simulink model "ES101A_DiagcMgr"  (R2013b)
settings: Solver=ode45  StartTime=0.0  StopTime=0.44  RelTol=1e-3
values from neighbouring files (symbols this model uses):
  BrdgVltg = DataDict.IpSignal    [ES101A_DiagcMgr_DataDict.m]
  DEM_CLEAR_PENDING = DataDict.Constant    [ES101A_DiagcMgr_DataDict.m]
  DEM_DTC_GROUP_ALL_DTCS = DataDict.Constant    [ES101A_DiagcMgr_DataDict.m]
  DFTAGICNTR_CNT_U08 = DataDict.Constant    [ES101A_DiagcMgr_DataDict.m]
  DIAGCMGR_NTCINFOSTSTESTFAILD_CNT_U08 = DataDict.Constant    [ES101A_DiagcMgr_DataDict.m]
  DIAGCMGR_NTCINFOSTSTESTFAILDTHISIGNCYC_CNT_U08 = DataDict.Constant    [ES101A_DiagcMgr_DataDict.m]
  DIAGCMGR_NTCINFOSTSTESTNOTCMPLTHISIGNCYC_CNT_U08 = DataDict.Constant    [ES101A_DiagcMgr_DataDict.m]
  DiagcMgrFltResp = DataDict.Calibration    [ES101A_DiagcMgr_DataDict.m]
  DiagcMgrNtcFltAry = DataDict.NVM    [ES101A_DiagcMgr_DataDict.m]
  DIAGCSTSCTRLDSHTDWNFLTPRSNT_CNT_U16 = DataDict.Constant    [ES101A_DiagcMgr_DataDict.m]
  DIAGCSTSDFTHWAG_CNT_U16 = DataDict.Constant    [ES101A_DiagcMgr_DataDict.m]
  DIAGCSTSDFTHWAGSERLCOMEXPRTVAL_CNT_U16 = DataDict.Constant    [ES101A_DiagcMgr_DataDict.m]
  DIAGCSTSDFTVEHSPD_CNT_U16 = DataDict.Constant    [ES101A_DiagcMgr_DataDict.m]
  DIAGCSTSININVAL_CNT_U16 = DataDict.Constant    [ES101A_DiagcMgr_DataDict.m]
  DIAGCSTSIVTR1INACTV_CNT_U16 = DataDict.Constant    [ES101A_DiagcMgr_DataDict.m]
  DIAGCSTSIVTR2INACTV_CNT_U16 = DataDict.Constant    [ES101A_DiagcMgr_DataDict.m]
  DIAGCSTSLIMDTPRFMNC_CNT_U16 = DataDict.Constant    [ES101A_DiagcMgr_DataDict.m]
  DIAGCSTSRAMPTOZEROFLTPRSNT_CNT_U16 = DataDict.Constant    [ES101A_DiagcMgr_DataDict.m]
  DIAGCSTSWHLIMBREJCTNDI_CNT_U16 = DataDict.Constant    [ES101A_DiagcMgr_DataDict.m]
  DTCIDXSTSFAIL_CNT_U08 = DataDict.Constant    [ES101A_DiagcMgr_DataDict.m]
  DTCIDXSTSNONTC_CNT_U08 = DataDict.Constant    [ES101A_DiagcMgr_DataDict.m]
  DTCIDXSTSNORES_CNT_U08 = DataDict.Constant    [ES101A_DiagcMgr_DataDict.m]
  DTCIDXSTSPASS_CNT_U08 = DataDict.Constant    [ES101A_DiagcMgr_DataDict.m]
  DTCIDXSTSUPDCFMD_CNT_U08 = DataDict.Constant    [ES101A_DiagcMgr_DataDict.m]
  ELECGLBPRM_IVTRCNT_CNT_U08 = DataDict.ConfigParam    [ES101A_DiagcMgr_DataDict.m]
  FLTINJ_DIAGCMGR_DIAGCSTSIVTR1INACTV = DataDict.Constant    [ES101A_DiagcMgr_DataDict.m]
  FLTINJ_DIAGCMGR_DIAGCSTSIVTR2INACTV = DataDict.Constant    [ES101A_DiagcMgr_DataDict.m]
  HwTq = DataDict.IpSignal    [ES101A_DiagcMgr_DataDict.m]
  IgnCntr = DataDict.IpSignal    [ES101A_DiagcMgr_DataDict.m]
  MAXDEBCNTRVAL_CNT_S16 = DataDict.Constant    [ES101A_DiagcMgr_DataDict.m]
  MAXRAMPRATE_ULSPERSEC_F32 = DataDict.Constant    [ES101A_DiagcMgr_DataDict.m]
  MINDEBCNTRVAL_CNT_S16 = DataDict.Constant    [ES101A_DiagcMgr_DataDict.m]
  MINRAMPRATE_ULSPERSEC_F32 = DataDict.Constant    [ES101A_DiagcMgr_DataDict.m]
  SCAMOTTQCMDTOONE_ULS_F32 = DataDict.Constant    [ES101A_DiagcMgr_DataDict.m]
  SCAMOTTQCMDTOZERO_ULS_F32 = DataDict.Constant    [ES101A_DiagcMgr_DataDict.m]
  SysSt = DataDict.IpSignal    [ES101A_DiagcMgr_DataDict.m]
  VehSpd = DataDict.IpSignal    [ES101A_DiagcMgr_DataDict.m]
undefined symbols (not defined in the file or in its folder): ActvMotTqCmdSca, ActvRampRate, AgiCntr, Dem_DTCFormatType, Dem_DTCOriginType, Dem_EventStatusType, DiagcData, DiagcMgrNtcMap, DiagcSts, DtcEnaMask, EcuT, HistNtcFltAry, MicroDiagcData, MotTq, NtcNr, NtcNrWithResd1, NtcStInfo, ProxySetNtcData, Sts, SysSt1, TOTNROFDTC_CNT_U08
libraries: simulink x151, FloatToFixd x5, NxtrNvM x4
(part 1 of 13)
settings Model: Creator=NZG49T  LastModifiedBy=nzg49t
settings DataIOCC: SaveFormat=Structure

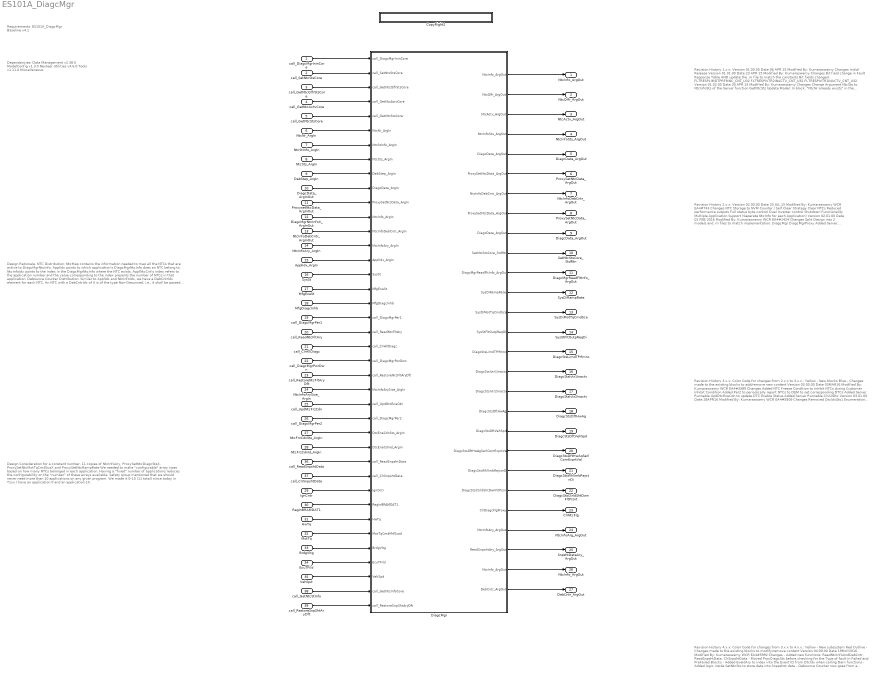
== system ES101A_DiagcMgr ==
  note: Revision History 1.x.x:
      |
      | Version		01.00.00
      | Date 		06 APR 15
      | Modified By: 	Kumaraswamy
      | Changes		Initial Release
      |
      | Version		01.01.00
      | Date 		23 APR 15
      | Modified By: 	Kumaraswamy
      | Changes		Bit field change in Fault Response Table AND update the .m file to match the constants
      | 			Bit fields changed: 	FLTRESPLIMDTPRFMNC_CNT_U32
      | 								FLTRESPIVTR2INACTV_CNT_U32
      | 								FLTRESPIVTR1INACTV_CNT_U32
      |
      | Version		01.02.00
      | Date 		30 APR 15
      | Modified By: 	Kumaraswamy
      | Changes		Change Argument NtcSts to NtcInfoSts of the Server function GetNtcSts
      | 			Update Model: In block, "NtcNr already exists" in the NtcFltAry when NTC fails, update the status byte
      | 			to show test failed bit as SET.
  note: Dependancies:
      |
      |    Data Management v2.38.0
      |    ModelConfig v1.3.0
      |    Nexteer Utilities v4.6.0
      |    Tools v1.11.0
      |    Miscellaneous
  note: Design Rationale:
      |
      | 	NTC Distribution:
      | 		NtcMap contains the information needed to map all the NTCs that are active to DiagcMgrNtcInfo.
      | 		ApplIdx points to which application's DiagcMgrNtcInfo does an NTC belong to.
      | 		NtcInfoIdx points to the index in the DiagcMgrNtcInfo where the NTC exists.
      | 		ApplNtcCnt's index refers to the application number and the value corresponding
      | 			to the index presents the number of NTCs in that application.
      |
      | 	Debounce Counter Distribution:
      | 		Similar to ApplIdx and NtcInfoIdx, we have a DebCntrIdx element for each NTC. An NTC with a DebCntrIdx of 0 is of the type Non-Deounced,
      | 		i.e., it shall be passed with SetNtcSts with NtcSts of either Passd or Faild only.
      | 		An NTC with a DebCntrIdx of Non-Zero is of the type Deounced, i.e., it shall be passed with SetNtcSts with NtcSts of either PrePassd or
      | 		PreFaild only.
      | 		Index 0 is used as a scratch pad for all the NTCs that are of the type Non-Debounced.
      |
      | 	NtcInfo for each application:
      | 		There will be a total of 11 DiagcMgrNtcInfo, one for each application.
      | 		If, for a specific program, we have 4 applications(say 0,3,4,10), each of these 4 applications with have certain number of NTCs in its respective
      | 		DiagcMgrNtcInfo(0,3,4,10). The rest of the DiagcMgrNtcInfo(1,2,5,6,7,8,9) will have just one element with the following default values:
      | 			AgiCntr:		255
      | 			Sts:			0
      | 			NtcStInfo:	0
      | 		Each application has its own array of structures that contains NTCs specific to its application.
      | 		The NTCs in any application will not be modified by any other application.
      |
      | 	DiagcSts, RampRate and Scale:
      | 		Each application will have a DiagcStsX, ProxyPerDiagcStsX and ProxySetNtcDiagcStsX (X is the application number):
      | 			DiagcStsX and ProxySetNtcDiagcStsX will be updated everytime the SetNtcSts function is called from the application.
      |
      | 			Each application makes a call to the DiagcMgrPer2 and clears the ProxyPerDiagcStsX and ProxySetNtcDiagcStsX.
      | 			DiagcMgrPer2 runs through all the NTCs in the application and updates the ProxyPerDiagcStsX with the most recent info
      | 			of all the NTCs that have failed this in this ignition cycle while ProxySetNtcDiagcStsX gets updated along with DiagcStsX
      | 			in the SetNtcSts function if any faults are set during the execution of DiagcMgrPer2.
      |
      | 			At the end of DiagcMgrPer2, DiagcStsX is  set equal to the ORed values of ProxyPerDiagcStsX and ProxySetNtcDiagcStsX
      |
      | 			DiagcMgrDiagcSts is the Word which stores the values that output the reduced performanc flags.
      | 			This value ORs all the DiagcStsX values and outputs the reduced performance flags in the DiagcMgrPer1.
      |
      | 			The same design rationale applies to RampRate  and Motor Torque Command Scale.
      | 			At the end of DiagcMgrPer2, RampRateX is  set to the MAX values of ProxyPerRampRateX and ProxySetNtcRampRateX.
      | 			At the end of DiagcMgrPer2, MotTqCmdScaX is  set to the MIN values of ProxyPerMotTqCmdScaX and ProxySetNtcMotTqCmdScaX.
      |
      | 	DiagcMgrInin:
      | 		DiagcMgrInin function shall be treated like server runnables by each application. An applicaiton shall call
      | 		DiagcMgrInin at initialization once passing the address of DiagcMgrNtcInfo to the DiagcMgr.
      |
      | 	DiagcMgrProxyPer1:
      | 		Each application will call DiagcMgrProxyPer1 at every 10ms interval passing the address of ProxySetNtcDiagcStsX. (X is the application number)
      | 		This is shown in DiagcMgrProxyX model.
      |
      | 	Model to SW Implementation:
      | 		Each NTC is mapped to only one of the DiagcMgrNtcInfo0 through 1DiagcMgrNtcInfo10 which will
      | 		be accessed by a pointer to the array of structure.
      | 		Model uses IF condition to look up the DiagcMgrNtcInfo (0 through 10) and uses the NtcInfoIdx to Index
      | 		into the NtcNr in the DiagcMgrNtcInfo.
      | 		SW implemention could involve using pointers to access the DiagcMgrNtcInfo (0 through 10) and use the
      | 		NtcInfoIdx to Index into the NtcNr in the DiagcMgrNtcInfo.
      |
      | 	Proxy Diagnostic Manager:
      | 		Each application will house a ProxyDiagnosticManager. Whenever a component inside an application calls
      | 		one of the server runnables, the ProxyDiagnosticManager makes a function call to the DiagcMgr and passes
      | 		some additional information of ApplIdx along with NtcNr, NtcSts, DebStep and NtcStInfo.
      |
      | 		The server runnables include DiagcMgrInit, SetNtcSts, GetNtcQlftSts, GetNtcActv and GetNtcSts.
      |
      | 	Handling Motor Control Interrrupts:
      | 		ES101A_v2_x_0 and above assumes that the Motor Control loop cannot set faults (call server runnables of DiagcMgr).
      |
      | 	Setting an NTC:
      | 		ES101A_v2_x_0 and above assumes that the same NTC Number cannot be set in mutilple loops
  note: Design Consideration for a constant number, 11 copies of NtcInfoAry, ProxySetNtcDiagcStsX, ProxySetNtcMotTqCmdScaX and ProxySetNtcRampRate
      |
      | We needed to make "configurable" array sizes based on how many NTCs belonged in each application.
      | Having a "fixed" number of applications reduces the configurability on the "number" of these arrays  available.
      | Safety group mentioned that we should never need more than 10 applications on any given program.
      | We made it 0-10 (11 total) since today in T1xx I have an application 0 and an application 10.
  note: Requirements:
      | ES101A_DiagcMgr Baseline v4.1
  note: Revision History 2.x.x:
      |
      | Version		02.00.00
      | Date 		20 JUL 15
      | Modified By: 	Kumaraswamy
      | WCR		EA4#743
      | Changes		NTC Storage to NVM
      | 			Counter / Self Clear Strategy
      | 			Clear NTCs
      | 			Reduced performance outputs
      | 			Full status byte control
      | 			Dual Inverter control
      | 			Shutdown Functionality
      | 			Multiple Application Support (Seperate NtcInfo for each Application)
      |
      | Version		02.01.00
      | Date 		02 FEB 2016
      | Modified By: 	Kumaraswamy
      | WCR		EA4#1424
      | Changes		Split Design into 2 models and .m files to match implementation:
      | 				DiagcMgr
      | 				DiagcMgrProxy
      | 			Added Server Runnables in DiagcMgr:
      | 				DiagcMgrIninCore
      | 				ClrAllNtc
      | 				RestoreNtcFltAryDft
      | 			Added Server Runnables in DiagcMgrProxy:
      | 				GetDiagcDataApplX
      | 				GetNtcInfoApplX
      | 			DiagcMgrActv Output is removed.
  note: Revision History 4.x.x:
      |
      | Color Code for changes from 3.x.x to 4.x.x.:
      | 	Yellow -  New subsystem
      | 	Red Outline -  Changes made to the existing blocks to modify/remove content
      |
      | Version		04.00.00
      | Date 		19MAY2016
      | Modified By: 	Kumaraswamy
      | WCR		EA4#5992
      | Changes		- Added new functions: ReadNtcInfoAndDebCntr, ReadSnpshtData, ClrSnpshtData
      | 			- Moved ProcDiagcSts before checking for the Type of fault in Failed and PreFailed Blocks
      | 			- Added EveIdAry to index into the Event ID from DtcIdx when calling Dem functions
      | 			- Added logic inside SetNtcSts to store data into Snapshot data
      | 			- Debounce Counter now goes from a negative value to DebStep if a Fail call is made to an NTC
      |
      | Version		04.01.00
      | Date 		16JUN2016
      | Modified By: 	Mohan
      | WCR		EA4#6355
      | Changes		- Added fault injection blocks in DiagcMgrPer1
      |
      | Version		04.02.00
      | Date 		21JUN2016
      | Modified By: 	Kumaraswamy
      | WCR		EA4#6360
      | Changes		- Changed call to the DEM: Clear all DTCs in DiagcMgrPer2
      | 			- Loop counter datatype changed from int32 to int16 in RestoreSnpshtAryDft
      | 			- RestoreSnpshtAryDft and RestoreNtcFltAryDft
      | 			- Changed argument SnpshtDataAry_ArgOut to ReadSnpshtAry_ArgOut of ReadSnpshtData Server Runnable
      | 			- Updated the GetNtcQlfrStsCore, GetNtcStsCore and GetNtcActvCore's default case
      | 			- Added client call GetNtcDebCntrAppIX to read the Debounce Counter of any NTC in any application
      | 			- Created a subgroup to create the snapshot bus to link to requirements
      |
      | Version		04.02.01
      | Date 		29JUN2016
      | Modified By: 	Kumaraswamy
      | WCR		EA4#6458
      | Changes		- Removed Data Type Convert blocks when loading 0s to NvM Block of SnpshtAry in RestoreSnpshtAryDft
      | 			- Added output out of the Default Case Switch Statement in Per2 for all NTCs
      | 			- Added a condition in If to check if DTC Idx is less than or equal to TOTNROFDTC_CNT_U08 in Per2
      | 			- ClrSnpshtData loaded with correct default values
      |
      | Version		04.03.00
      | Date 		15AUG2016
      | Modified By: 	Kumaraswamy
      | WCR		EA4#6904
      | Changes		- PIL Optimizations
      |
      | Version		04.04.00
      | Date 		14SEP2016
      | Modified By: 	Kumaraswamy
      | WCR		EA4#7573
      | Changes		- Overflow condition averted by adding logic in "if condition" inside PreFaild
      | 			- Added logic to return a 0 value of DebCntr for Non Debounced NTCs in the ReadNtcInfoAndDebCntr server runnable
      | 			since all Non Debounced NTCs use the DebCntrIdx of 0 as a scratchpad
      |
      | Version		04.05.00
      | Date 		15NOV2016
      | Modified By: 	Kumaraswamy
      | WCR		EA4#8249
      | Changes		- UpdSnpshtData  logic updated to prevent multiple entries of same NTC being set
      | 			- Added logic to call UpdSnpshtData only once if the NTC transitions from Pass to Fail
      |
      | Version		04.06.00
      | Date 		01DEC2016
      | Modified By: 	Kumaraswamy
      | WCR		EA4#8667
      | Changes		- Added write to Set Ram Block Status in ClrSnpshtData  function after the for loop
  note: Revision History 3.x.x:
      |
      | Color Code for changes from 2.x.x to 3.x.x.:
      | 	Yellow -  New blocks
      | 	Blue -  Changes made to the existing blocks to add/remove new content
      |
      | Version		03.00.00
      | Date 		03MAR16
      | Modified By: 	Kumaraswamy
      | WCR		EA4#3389
      | Changes
      | 			Added NTC Freeze Condition to Inhibit NTCs during Customer Inhibit Condition
      | 			Added Per2 to periodically report NTCs to DEM to set corresponding DTCs
      | 			Added Server Runnable UpdDtcEnaCdn to update DTC Enable Status
      | 			Added Server Runnable ClrAllDtc
      |
      | Version		03.01.00
      | Date 		28APR16
      | Modified By: 	Kumaraswamy
      | WCR		EA4#5509
      | Changes		Removed DtcIdxSts1 Enumeration and replaced it's members with constants since it is used
      | 			only by temp variables
      | 			ReadNtcFltAry's output argument renamed correctly as per .m file
      | 			Comments updated
      | 			Added PIM PrevClrDiagcFlag in the .m file
      |
      | Version		03.02.00
      | Date 		29APR16
      | Modified By: 	Kumaraswamy
      | WCR		EA4#5509
      | Changes		Initialized DtcIdxCurrSts 0th element in the Initialization of Per2
      | 			Matched the PrevClrDtcFlg, ClrDtcFlg, ClrDiagcFlgProxy, PrevClrNtcFlgX to have a DataType of Boolean in .m file
      | 			UpdDtcEnaCdn changed from Rte to NonRte
      |
      | Version		03.03.00
      | Date 		26MAY16
      | Modified By: 	Kumaraswamy
      | WCR		EA4#5907
      | Changes		Updated the description of DtcEnaMask to show the length of the array.
  call_DiagcMgrIninCore : Inport
  call_SetNtcStsCore : Inport  Port=2
  call_GetNtcQlfrStsCore : Inport  RequirementInfo={} %GIDa_139edafb_ed2e_4817_b523_bf8478521829  Port=3
  call_GetNtcActvCore : Inport  Port=4
  call_GetNtcStsCore : Inport  Port=5
  NtcNr_ArgIn : Inport  Port=6
  NtcStInfo_ArgIn : Inport  Port=7
  NtcSts_ArgIn : Inport  Port=8
  DebStep_ArgIn : Inport  Port=9
  DiagcData_ArgInOut : Inport  Port=10
  ProxysetNtcData_ArgInOut : Inport  RequirementInfo={} %GIDa_51b0a352_6025_4132_85e8_dce6b37dec3f  Port=11
  DiagcMgrNtcInfoX_ArgInOut : Inport  Port=12
  NtcInfoDebCntr_ArgInOut : Inport  Port=13
  NtcInfoAry_ArgIn : Inport  Port=14
  ApplIdx_ArgIn : Inport  Port=15
  SysSt : Inport  Port=16
  MfgEnaSt : Inport  Port=17
  MfgDiagcInhb : Inport  RequirementInfo="{'linktype_rmi_doors' '0000c474 (/ESG Group/FDD Module Requirements/EA4 Specific/ES101A_DiagcMgr)' '#ES101A_301' 'true' 'REQ:  ES101A_301' '' } %GIDa_f9f3ee9e_ad90_4a3f_b3fd_4c7a6708a1f3"  Port=18
  call_DiagcMgrPer1 : Inport  Port=19
  call_ReadNtcFltAry : Inport  Port=20
  call_ClrAllDiagc : Inport  Port=21
  call_DiagcMgrPwrDwn : Inport  Port=22
  call_RestoreNtcFltAryDft : Inport  Port=23
  NtcInfoArySize_ArgIn : Inport  Port=24
  call_UpdNtcFrzCdn : Inport  Port=25
  call_DiagcMgrPer2 : Inport  Port=26
  NtcFrzCdnSts_ArgIn : Inport  Port=27
  NtcFrzCdnId_ArgIn : Inport  Port=28
  IgnCntr : Inport  Port=29
  RegInBRAMDAT1 : Inport  Port=30
  HwTq : Inport  Port=31
  MotTq : Inport  Port=32
  BrdgVltg : Inport  Port=33
  EcuTFild : Inport  Port=34
  VehSpd : Inport  Port=35
  call_ReadSnpshtData : Inport  Port=36
  call_ClrSnpshtData : Inport  Port=37
  call_GetNtcStInfo : Inport  Port=38
  call_RestoreSnpShtAryDft : Inport  Port=39
  CopyRight2 : Subsystem  Description=|  mask(Copyright Information){none=on}
      | Copyright info block.                                               
      |                                                                     
      | Place copyright information at the top of every subsystem in design.
      mask prompts: none "No parameters"
      mask help: Place copyright information at the top of every subsystem in design.
      mask Display:
      | NxtrConf = 'Nexteer Confidential';
      | 
      | sys = bdroot; %handle for the current model ("system")
      | first = get_param(sys,'Created');
      | first = first(end-3:end);  %year is last four digits
      | 
      | last = get_param(sys,'LastModifiedDate');
      | if isempty(last)
      |     last = datestr(now,'yyyy');
      | else
      |     last = last(end-3:end);
      | end
      | 
      | if strcmp(first,last)
      |     fprintf('%s -- Copyright %s Nexteer',NxtrConf,first)
      | else
      |     fprintf('%s -- %s%s- %s Nexteer',NxtrConf,char(169),first,last)
      | end
  DiagcMgr : Subsystem
  "NtcInfo_ArgOut " : Outport
  NtcQlfr_ArgOut : Outport  Port=2
  NtcActv_ArgOut : Outport  Port=3
  NtcInfoSts_ArgOut : Outport  Port=4
  "DiagcData_ArgOut " : Outport  Port=5
  "ProxySetNtcData_ArgOut " : Outport  Port=6
  "NtcInfoDebCntr_ArgOut " : Outport  Port=7
  ProxySetNtcData_ArgOut : Outport  Port=8
  DiagcData_ArgOut : Outport  Port=9
  SetNtcStsCore_StdRtn : Outport  Port=10
  DiagcMgrReadFltInfo_ArgOut : Outport  Port=11
  SysDiRampRate : Outport  Port=12
  SysDiMotTqCmdSca : Outport  Port=13
  SysStFltOutpReqDi : Outport  Port=14
  DiagcStsLimdTPrfmnc : Outport  Port=15
  DiagcStsIvtr1Inactv : Outport  Port=16
  DiagcStsIvtr2Inactv : Outport  Port=17
  DiagcStsDftHwAg : Outport  Port=18
  DiagcStsDftVehSpd : Outport  Port=19
  DiagcStsDftHwAgSerlComExprtVal : Outport  Port=20
  DiagcStsWhlImbRejctnDi : Outport  Port=21
  DiagcStsCtrldShtDwnFltPrsnt : Outport  Port=22
  ClrNtcFlg : Outport  Port=23
  NtcInfoArg_ArgOut : Outport  Port=24
  SnpshtDataAry_ArgOut : Outport  Port=25
  NtcInfo_ArgOut : Outport  Port=26
  DebCntr_ArgOut : Outport  Port=27
  wires:
  SysSt/1 -> DiagcMgr/16(SysSt)
  MfgEnaSt/1 -> DiagcMgr/17(MfgEnaSt)
  MfgDiagcInhb/1 -> DiagcMgr/18(MfgDiagcInhb)
  call_DiagcMgrPer1/1 -> DiagcMgr/19(call_DiagcMgrPer1)
  call_ReadNtcFltAry/1 -> DiagcMgr/20(call_ReadNtcFltAry)
  call_DiagcMgrPwrDwn/1 -> DiagcMgr/22(call_DiagcMgrPwrDwn)
  DiagcMgr/12(SysDiRampRate) -> SysDiRampRate/1
  DiagcMgr/13(SysDiMotTqCmdSca) -> SysDiMotTqCmdSca/1
  DiagcMgr/17(DiagcStsIvtr2Inactv) -> DiagcStsIvtr2Inactv/1
  DiagcMgr/14(SysStFltOutpReqDi) -> SysStFltOutpReqDi/1
  DiagcMgr/15(DiagcStsLimdTPrfmnc) -> DiagcStsLimdTPrfmnc/1
  DiagcMgr/16(DiagcStsIvtr1Inactv) -> DiagcStsIvtr1Inactv/1
  DiagcMgr/20(DiagcStsDftHwAgSerlComExprtVal) -> DiagcStsDftHwAgSerlComExprtVal/1
  DiagcMgr/18(DiagcStsDftHwAg) -> DiagcStsDftHwAg/1
  DiagcMgr/19(DiagcStsDftVehSpd) -> DiagcStsDftVehSpd/1
  DiagcMgr/21(DiagcStsWhlImbRejctnDi) -> DiagcStsWhlImbRejctnDi/1
  DiagcMgr/22(DiagcStsCtrldShtDwnFltPrsnt) -> DiagcStsCtrldShtDwnFltPrsnt/1
  call_ClrAllDiagc/1 -> DiagcMgr/21(call_ClrAllDiagc)
  DiagcMgr/11(DiagcMgrReadFltInfo_ArgOut) -> DiagcMgrReadFltInfo_ArgOut/1
  DiagcMgr/23(ClrDiagcFlgProxy) -> ClrNtcFlg/1
  call_RestoreNtcFltAryDft/1 -> DiagcMgr/23(call_RestoreNtcFltAryDft)
  call_GetNtcStsCore/1 -> DiagcMgr/5(call_GetNtcStsCore)
  NtcNr_ArgIn/1 -> DiagcMgr/6(NtcNr_ArgIn)
  call_SetNtcStsCore/1 -> DiagcMgr/2(call_SetNtcStsCore)
  call_GetNtcQlfrStsCore/1 -> DiagcMgr/3(call_GetNtcQlfrStsCore)
  call_DiagcMgrIninCore/1 -> DiagcMgr/1(call_DiagcMgrIninCore)
  NtcStInfo_ArgIn/1 -> DiagcMgr/7(NtcStInfo_ArgIn)
  call_GetNtcActvCore/1 -> DiagcMgr/4(call_GetNtcActvCore)
  NtcSts_ArgIn/1 -> DiagcMgr/8(NtcSts_ArgIn)
  DiagcData_ArgInOut/1 -> DiagcMgr/10(DiagcData_ArgIn)
  NtcInfoAry_ArgIn/1 -> DiagcMgr/14(NtcInfoAry_ArgIn)
  DebStep_ArgIn/1 -> DiagcMgr/9(DebStep_ArgIn)
  ProxysetNtcData_ArgInOut/1 -> DiagcMgr/11(ProxySetNtcData_ArgIn)
  DiagcMgrNtcInfoX_ArgInOut/1 -> DiagcMgr/12(NtcInfo_ArgIn)
  NtcInfoDebCntr_ArgInOut/1 -> DiagcMgr/13(NtcInfoDebCntr_ArgIn)
  ApplIdx_ArgIn/1 -> DiagcMgr/15(ApplIdx_ArgIn)
  NtcInfoArySize_ArgIn/1 -> DiagcMgr/24(NtcInfoArySize_ArgIn)
  DiagcMgr/5("DiagcData_ArgOut ") -> "DiagcData_ArgOut "/1
  DiagcMgr/2(NtcQlfr_ArgOut) -> NtcQlfr_ArgOut/1
  DiagcMgr/9(DiagcData_ArgOut) -> DiagcData_ArgOut/1
  DiagcMgr/4(NtcInfoSts_ArgOut) -> NtcInfoSts_ArgOut/1
  DiagcMgr/10(SetNtcStsCore_StdRtn) -> SetNtcStsCore_StdRtn/1
  DiagcMgr/8(ProxySetNtcData_ArgOut) -> ProxySetNtcData_ArgOut/1
  DiagcMgr/7("NtcInfoDebCntr_ArgOut ") -> "NtcInfoDebCntr_ArgOut "/1
  DiagcMgr/1("NtcInfo_ArgOut ") -> "NtcInfo_ArgOut "/1
  DiagcMgr/3(NtcActv_ArgOut) -> NtcActv_ArgOut/1
  DiagcMgr/6("ProxySetNtcData_ArgOut ") -> "ProxySetNtcData_ArgOut "/1
  DiagcMgr/24(NtcInfoAry_ArgOut) -> NtcInfoArg_ArgOut/1
  NtcFrzCdnId_ArgIn/1 -> DiagcMgr/28(DtcEnaCdnId_ArgIn)
  call_DiagcMgrPer2/1 -> DiagcMgr/26(call_DiagcMgrPer2)
  NtcFrzCdnSts_ArgIn/1 -> DiagcMgr/27(DtcEnaCdnSts_ArgIn)
  call_UpdNtcFrzCdn/1 -> DiagcMgr/25(call_UpdDtcEnaCdn)
  DiagcMgr/25(ReadSnpshtAry_ArgOut) -> SnpshtDataAry_ArgOut/1
  IgnCntr/1 -> DiagcMgr/31(IgnCntr)
  RegInBRAMDAT1/1 -> DiagcMgr/32(RegInBRAMDAT1)
  HwTq/1 -> DiagcMgr/33(HwTq)
  MotTq/1 -> DiagcMgr/34(MotTqCmdMrfScad)
  BrdgVltg/1 -> DiagcMgr/35(BrdgVltg)
  EcuTFild/1 -> DiagcMgr/36(EcuTFild)
  VehSpd/1 -> DiagcMgr/37(VehSpd)
  call_ReadSnpshtData/1 -> DiagcMgr/29(call_ReadSnpshtData)
  call_ClrSnpshtData/1 -> DiagcMgr/30(call_ClrSnpshtData)
  DiagcMgr/26(NtcInfo_ArgOut) -> NtcInfo_ArgOut/1
  call_GetNtcStInfo/1 -> DiagcMgr/38(call_GetNtcInfoCore)
  DiagcMgr/27(DebCntr_ArgOut) -> DebCntr_ArgOut/1
  call_RestoreSnpShtAryDft/1 -> DiagcMgr/39(call_RestoreSnpShtAryDft)

== system ES101A_DiagcMgr/CopyRight2 ==

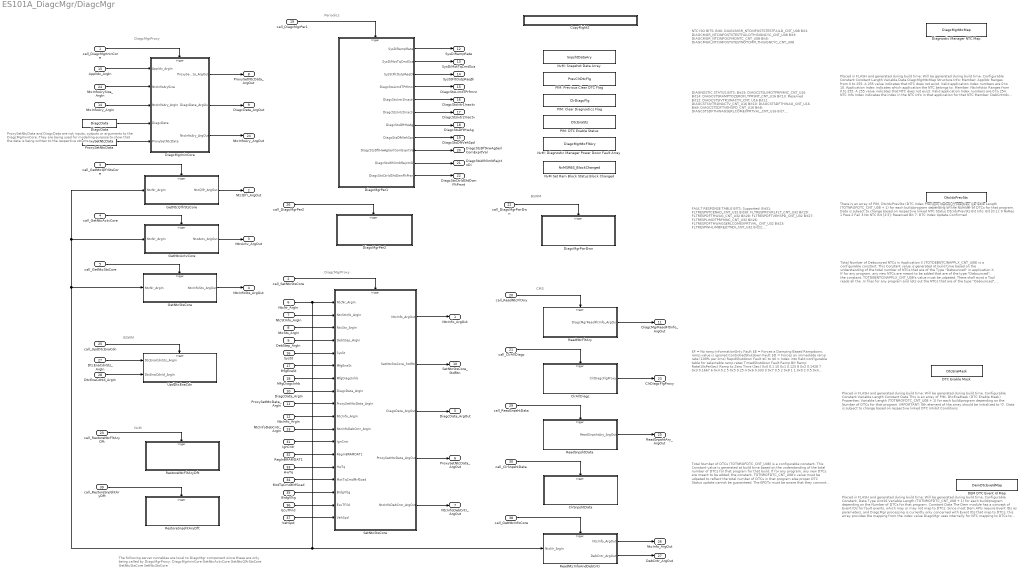
== system ES101A_DiagcMgr/DiagcMgr ==
  note: NvM
  note: Total Number of Debounced NTCs in Application X (TOTDEBNTCINAPPLX_CNT_U08)
      | is a configurable constant.
      |
      | This Constant value is generated at build time based on the understanding of
      | the total number of NTCs that are of the Type "Debounced" in application X.
      |
      | If for any program, any new NTCs are meant to be added that are of the type
      | "Debounced", the constant, TOTDEBNTCINAPPLX_CNT_U08's value must be udpated.
      |
      | There shall exist a Tool reads all the .m files for any program and lists out the NTCs that
      | are of the type "Debounced".
      |
      | The integrator shall use the tool to get this info and update the constant's value.
  note: The following server runnables are local to DiagcMgr component since these are
      | only being called by DiagcMgrProxy:
      |
      | 	DiagcMgrIninCore
      | 	GetNtcActvCore
      | 	GetNtcQlfrStsCore
      | 	GetNtcStsCore
      | 	SetNtcStsCore
  note: Placed in FLASH and generated during build time:
      | Will be generated during build time.
      | Configurable Constant
      | Constant Length
      | Variable Data
      |
      | 	DiagcMgrNtcMap Structure Info:
      | 		Member: ApplIdx
      | 			Ranges from 0 to 255.
      | 			A 255 value indicates that NTC does not exist.
      | 			Valid application Index numbers are 0 to 10.
      | 			Application Index indicates which application the NTC belongs to.
      |
      | 		Member: NtcInfoIdx
      | 			Ranges from 0 to 255.
      | 			A 255 value indicates that NTC does not exist.
      | 			Valid application Index numbers are 0 to 254.
      | 			NTC Info Index indicates the index in the NTC Info in that application for that NTC
      |
      | 		Member: DebCntrIdx
      | 			Ranges from 0 to TOTDEBNTCINAPPLX_CNT_U08 + 1.
      | 			A 0 value indicates that NTC does not have a Debounce Counter.
      | 			The counter at index 0 has no significance. It is only to make design simpler.
      | 			Valid application Index numbers are 1 to TOTDEBNTCINAPPLX_CNT_U08 + 1.
      | 			Debounce Counter Index indicates which application the NTC belongs to.
  note: FAULT  RESPONSE  TABLE  BITS:
      |
      | Supported:
      | 	Bit31: FLTRESPNTCENAD_CNT_U32
      | 	Bit30: FLTRESPRCVRLFLT_CNT_U32
      | 	Bit29: FLTRESPDFTHWAG_CNT_U32
      | 	Bit28: FLTRESPDFTVEHSPD_CNT_U32
      | 	Bit27: FLTRESPLIMDTPRFMNC_CNT_U32
      | 	Bit26: FLTRESPDFTHWAGSERLCOMEXPRTVAL_CNT_U32
      | 	Bit23: FLTRESPWHLIMBREJCTNDI_CNT_U32
      | 	Bit22: FLTRESPSNPSHTDATAENAD_CNT_U32*
      | 	Bit16: FLTRESPIVTR2INACTV_CNT_U32
      | 	Bit15: FLTRESPIVTR1INACTV_CNT_U32
      | 	Bit14: FLTRESPMFGINHBINENAST_CNT_U32
      | 	Bit13: FLTRESPMFGINHBNOTINENAST_CNT_U32
      |  	Bit12: FLTRESPSTSLOCKDTHISIGNCYC_CNT_U32
      | 	Bit11: FLTRESPRAMPBITS_CNT_U32
      | 	Bit10: FLTRESPRAMPBITS_CNT_U32
      | 	Bit09: FLTRESPRAMPBITS_CNT_U32
      | 	Bit08: FLTRESPRAMPBITS_CNT_U32
      | 	Bit07: FLTRESPDTCIDX_CNT_U32
      | 	Bit06: FLTRESPDTCIDX_CNT_U32
      | 	Bit05: FLTRESPDTCIDX_CNT_U32
      | 	Bit04: FLTRESPDTCIDX_CNT_U32
      | 	Bit03: FLTRESPDTCIDX_CNT_U32
      | 	Bit02: FLTRESPDTCIDX_CNT_U32
      | 	Bit01: FLTRESPDTCIDX_CNT_U32
      | 	Bit00: FLTRESPDTCIDX_CNT_U32
      |
      | * Newly Added
  note: NTC  ISO  BITS:
      |
      | Bit0: DIAGCMGR_NTCINFOSTSTESTFAILD_CNT_U08
      | Bit1: DIAGCMGR_NTCINFOSTSTESTFAILDTHISIGNCYC_CNT_U08
      | Bit3: DIAGCMGR_NTCINFOCFMDNTC_CNT_U08
      | Bit6: DIAGCMGR_NTCINFOSTSTESTNOTCMPLTHISIGNCYC_CNT_U08
  note: DIAGNOSTIC  STATUS  BITS:
      |
      | Bit15: DIAGCSTSLIMDTPRFMNC_CNT_U16
      | Bit14: DIAGCSTSRAMPTOZEROFLTPRSNT_CNT_U16
      | Bit13: Reserved
      | Bit12: DIAGCSTSIVTR1INACTV_CNT_U16
      | Bit11: DIAGCSTSIVTR2INACTV_CNT_U16
      | Bit10: DIAGCSTSDFTHWAG_CNT_U16
      | Bit9:   DIAGCSTSDFTVEHSPD_CNT_U16
      | Bit8:   DIAGCSTSDFTHWAGSERLCOMEXPRTVAL_CNT_U16
      | Bit7:   DIAGCSTSWHLIMBREJCTNDI_CNT_U16
      | Bit6:	   DIAGCSTSCTRLDSHTDWNFLTPRSNT_CNT_U16
  note: $F = No ramp
      | 	InformationOnly Fault
      | $E = Forces a Damping Based Rampdown, ramp value is ignored
      | 	ControlledShutdown Fault
      | $D = Forces an immediate ramp rate (100% per 2ms)
      | 	RapidShutdown Fault
      | $C to $0 = Index into field configurable table for selectable ramp rates
      | 	TimedShutdown Fault
      |
      | Ramp Bit	Ramp Rate(UlsPerSec)	Ramp to Zero Time (Sec)
      | 0x0			0.1						10
      | 0x1			0.125					8
      | 0x2			0.1428					7
      | 0x3			0.1667					6
      | 0x4			0.2						5
      | 0x5			0.25						4
      | 0x6			0.333					3
      | 0x7			0.5						2
      | 0x8			1						1
      | 0x9			2						0.5
      | 0xA			3.333					0.3
      | 0xB			10						0.1
      | 0xC			500						0.002
  note: ProxySetNtcData and DiagcData
      | are not inputs, outputs or arguments to the
      | DiagcMgrIninCore. They are being used for
      | modelling purpose to show that the data is
      | being written to the respective structs.
  note: There is an array of PIM, DtcIdxPrevSts (DTC Index Previous Status)
      | 	Properties:
      | 		Variable Length (TOTNROFDTC_CNT_U08 + 1) for each build/program
      | 		depending on the Number of DTCs for that program.
      | 		Data is subject to change based on respective linked NTC Status
      |
      | 	DtcIdxPrevSts Bit Info:
      | 		Bit [0:1]:
      | 		0 NoRes
      | 		1 Pass
      | 		2 Fail
      | 		3 No NTC
      |
      | 		Bit [2:5]:
      | 		Reserved
      |
      | 		Bit 7:
      | 		DTC Index Update Confirmed
  note: Placed in FLASH and generated during build time:
      | Will be generated during build time.
      | Configurable Constant
      | Variable Length
      | Constant Data
      |
      | 	This is an array of PIM, DtcEnaMask (DTC  Enable Mask)
      | 	Properties:
      | 		Variable Length (TOTNROFDTC_CNT_U08 + 1) for each build/program depending
      | 		on the Number of DTCs for that program.
      |
      | 		IMPORTANT: 0th element of the array should be initialized to '0'.
      |
      | 		Data is subject to change based on respective linked DTC Inhibit Conditions
  note: Total Number of DTCs (TOTNROFDTC_CNT_U08) is a configurable
      | constant.
      |
      | This Constant value is generated at build time based on the understanding of
      | the total number of DTCs for that program for that build.
      | If for any program, any new DTCs are meant to be added, the constant,
      | TOTNROFDTC_CNT_U08's value must be udpated to reflect the total
      | number of DTCs in that program else proper DTC Status update cannot be
      | guaranteed.
      | The EPDTs must be aware that they cannont add new DTC numbers just
      | by changing the calibration, FltRespTbl.
      |
      | The EPDT shall inform the Integrator to inform them the total number of
      | DTCs in the program.
      | OR
      | The integrator shall ask the EPDT to get this info and update the constant.
  note: Placed in FLASH and generated during build time:
      | 	Will be generated during build time.
      | 	Configurable Constant, Data Type Uint16
      | 	Variable Length (TOTNROFDTC_CNT_U08 + 1) for each build/program depending on the Number of DTCs
      | 	for that program.
      | 	Constant Data
      |
      |
      |
      |
      | The Dem module has a concept of Event IDs for fault events, which may or may not map to DTCs.
      | Since most Dem APIs require Event IDs as parameters, and DiagcMgr processing is currently only concerned with Event IDs
      | that map to DTCs, this array provides the mapping from the index value DiagcMgr uses internally for NTC mapping to DTCs to
      | the Event ID that the Dem identifies for a particular DTC. This table is required because the ordering the Dem uses does not
      | guarantee that Event IDs that are mapped to DTCs are always places consecutively.
  note: BSWM
  note: DiagcMgrProxy
  note: DiagcMgrProxy
  note: CMS
  note: BSWM
  note: Periodics
  call_DiagcMgrIninCore : Inport
  call_SetNtcStsCore : Inport  Port=2
  call_GetNtcQlfrStsCore : Inport  Port=3
  call_GetNtcActvCore : Inport  Port=4
  call_GetNtcStsCore : Inport  Port=5
  NtcNr_ArgIn : Inport  Port=6  OutDataTypeStr=Enum: NtcNr1
  NtcStInfo_ArgIn : Inport  Port=7
  NtcSts_ArgIn : Inport  Port=8
  DebStep_ArgIn : Inport  Port=9
  DiagcData_ArgIn : Inport  Port=10
  ProxySetNtcData_ArgIn : Inport  Port=11
  NtcInfo_ArgIn : Inport  Port=12
  NtcInfoDebCntr_ArgIn : Inport  Port=13
  NtcInfoAry_ArgIn : Inport  Port=14
  ApplIdx_ArgIn : Inport  Port=15
  SysSt : Inport  Port=16
  MfgEnaSt : Inport  Port=17
  MfgDiagcInhb : Inport  Port=18
  call_DiagcMgrPer1 : Inport  Port=19
  call_ReadNtcFltAry : Inport  Port=20
  call_ClrAllDiagc : Inport  Port=21
  call_DiagcMgrPwrDwn : Inport  Port=22
  call_RestoreNtcFltAryDft : Inport  Port=23
  NtcInfoArySize_ArgIn : Inport  Port=24
  call_UpdDtcEnaCdn : Inport  Port=25
  call_DiagcMgrPer2 : Inport  Port=26
  DtcEnaCdnSts_ArgIn : Inport  Port=27
  DtcEnaCdnId_ArgIn : Inport  Port=28
  call_ReadSnpshtData : Inport  Port=29
  call_ClrSnpshtData : Inport  Port=30
  IgnCntr : Inport  Port=31
  RegInBRAMDAT1 : Inport  Port=32
  HwTq : Inport  Port=33
  MotTqCmdMrfScad : Inport  Port=34
  BrdgVltg : Inport  Port=35
  EcuTFild : Inport  Port=36
  VehSpd : Inport  Port=37
  call_GetNtcInfoCore : Inport  Port=38
  call_RestoreSnpShtAryDft : Inport  Port=39
  ClrAllDiagc : Subsystem  RequirementInfo="{'linktype_rmi_doors' '0000c474 (/ESG Group/FDD Module Requirements/EA4 Specific/ES101A_DiagcMgr)' '#ES101A_285' 'true' 'REQ:  ES101A_285' '' ; 'linktype_rmi_doors' '0000c474 (/ESG Group/FDD Module Requirements/EA4 Specific/ES101A_DiagcMgr)' '#ES101A_318' 'true' 'REQ:  ES101A_318' '' ; 'linktype_rmi_doors' '0000c474 (/ESG Group/FDD Module Requirements/EA4 Specific/ES101A_DiagcMgr)' '#ES101A_319' 'true' 'REQ:  ES101A_319' '' } %GIDa_0ae01384_136e_461f_80db_32dc1ddeed9a"
  ClrSnpshtData : Subsystem  RequirementInfo="{'linktype_rmi_doors' '0000c474 (/ESG Group/FDD Module Requirements/EA4 Specific/ES101A_DiagcMgr)' '#ES101A_334' 'true' 'REQ:  ES101A_334' '' } %GIDa_c6db68a1_d681_4345_964e_f921ff52ec9e"
      settings: AttributesFormatString=%<Description>
  CopyRight2 : Subsystem  Description=|  mask(Copyright Information){none=on}
      | Copyright info block.                                               
      |                                                                     
      | Place copyright information at the top of every subsystem in design.
      mask prompts: none "No parameters"
      mask help: Place copyright information at the top of every subsystem in design.
      mask Display:
      | NxtrConf = 'Nexteer Confidential';
      | 
      | sys = bdroot; %handle for the current model ("system")
      | first = get_param(sys,'Created');
      | first = first(end-3:end);  %year is last four digits
      | 
      | last = get_param(sys,'LastModifiedDate');
      | if isempty(last)
      |     last = datestr(now,'yyyy');
      | else
      |     last = last(end-3:end);
      | end
      | 
      | if strcmp(first,last)
      |     fprintf('%s -- Copyright %s Nexteer',NxtrConf,first)
      | else
      |     fprintf('%s -- %s%s- %s Nexteer',NxtrConf,char(169),first,last)
      | end
  DEM DTC Event Id Map : DataStoreMemory  DataStoreName=DemDtcEveIdMap  InitialValue=[0 0 0 0 0 0 0 0 0 0 0 0 0 0 0 0 0 0 0 0 0 0 0 0 0 0 0 0 0]  OutDataTypeStr=uint16  StateMustResolveToSignalObject=on
  DTC Enable Mask : Constant  Value=DtcEnaMask
  DiagcData : Constant  Value=DiagcData
  DiagcMgrIninCore : Subsystem  RequirementInfo={} %GIDa_c32d5ffc_be28_4486_b8ca_7aefc7896ac2
      settings: AttributesFormatString=%<Description>
  DiagcMgrPer1 : Subsystem  Description=|  RequirementInfo="{'linktype_rmi_doors' '0000c474 (/ESG Group/FDD Module Requirements/EA4 Specific/ES101A_DiagcMgr)' '#ES101A_265' 'true' 'REQ:  ES101A_265' '' ; 'linktype_rmi_doors' '0000c474 (/ESG Group/FDD Module Requirements/EA4 Specific/ES101A_DiagcMgr)' '#ES101A_263' 'true' 'REQ:  ES101A_263' '' ; 'linktype_rmi_doors' '0000c474 (/ESG Group/FDD Module Requirements/EA4 Specific/ES101A_DiagcMgr)' '#ES101A_260' 'true' 'REQ:  ES101A_260' '' ; 'linktype_rmi_doors' '0000c474 (/ESG Group/FDD Module Requirements/EA4 Specific/ES101A_DiagcMgr)' '#ES101A_261' 'true' 'REQ:  ES101A_261' '' ; 'linktype_rmi_doors' '0000c474 (/ESG Group/FDD Module Requirements/EA4 Specific/ES101A_DiagcMgr)' '#ES101A_258' 'true' 'REQ:  ES101A_258' '' ; 'linktype_rmi_doors' '0000c474 (/ESG Group/FDD Module Requirements/EA4 Specific/ES101A_DiagcMgr)' '#ES101A_81' 'true' 'REQ:  ES101A_81' '' ; 'linktype_rmi_doors' '0000c474 (/ESG Group/FDD Module Requirements/EA4 Specific/ES101A_DiagcMgr)' '#ES101A_202' 'true' 'REQ:  ES101A_202' '' ; 'linktype_rmi_doors' '0000c474 (/ESG Group/FDD Module Requirements/EA4 Specific/ES101A_DiagcMgr)' '#ES101A_204' 'true' 'REQ:  ES101A_204' '' ; 'linktype_rmi_doors' '0000c474 (/ESG Group/FDD Module Requirements/EA4 Specific/ES101A_DiagcMgr)' '#ES101A_86' 'true' 'REQ:  ES101A_86' '' ; 'linktype_rmi_doors' '0000c474 (/ESG Group/FDD Module Requirements/EA4 Specific/ES101A_DiagcMgr)' '#ES101A_289' 'true' 'REQ:  ES101A_289' '' ; 'linktype_rmi_doors' '0000c474 (/ESG Group/FDD Module Requirements/EA4 Specific/ES101A_DiagcMgr)' '#ES101A_208' 'true' 'REQ:  ES101A_208' '' ; 'linktype_rmi_doors' '0000c474 (/ESG Group/FDD Module Requirements/EA4 Specific/ES101A_DiagcMgr)' '#ES101A_292' 'true' 'REQ:  ES101A_292' '' ; 'linktype_rmi_doors' '0000c474 (/ESG Group/FDD Module Requirements/EA4 Specific/ES101A_DiagcMgr)' '#ES101A_77' 'true' 'REQ:  ES101A_77' '' } %GIDa_52e42c1b_cb7c_42fe_8893_73dda9bc1548"
      | 2ms
      | Update Outputs
      settings: AttributesFormatString=%<Description>
  DiagcMgrPer2 : Subsystem  Description=100ms  RequirementInfo="{'linktype_rmi_doors' '0000c474 (/ESG Group/FDD Module Requirements/EA4 Specific/ES101A_DiagcMgr)' '#ES101A_322' 'true' 'REQ:  ES101A_322' '' } %GIDa_75412a4c_0f46_451b_9dd4_c7cc359f90f7"
      settings: AttributesFormatString=%<Description>
  DiagcMgrPwrDwn : Subsystem  RequirementInfo="{'linktype_rmi_doors' '0000c474 (/ESG Group/FDD Module Requirements/EA4 Specific/ES101A_DiagcMgr)' '#ES101A_197' 'true' 'REQ:  ES101A_197' '' ; 'linktype_rmi_doors' '0000c474 (/ESG Group/FDD Module Requirements/EA4 Specific/ES101A_DiagcMgr)' '#ES101A_248' 'true' 'REQ:  ES101A_248' '' ; 'linktype_rmi_doors' '0000c474 (/ESG Group/FDD Module Requirements/EA4 Specific/ES101A_DiagcMgr)' '#ES101A_249' 'true' 'REQ:  ES101A_249' '' ; 'linktype_rmi_doors' '0000c474 (/ESG Group/FDD Module Requirements/EA4 Specific/ES101A_DiagcMgr)' '#ES101A_217' 'true' 'REQ:  ES101A_217' '' } %GIDa_6ab14065_fee4_408b_9398_b5d7cfe2e3ff"
      settings: AttributesFormatString=%<Description>
  Diagnostic Manager NTC Map : DataStoreMemory  Description=FOR SIMULATION ONLY!  RequirementInfo={} %GIDa_20708300_7b30_482c_83ee_957e7e398e3c  DataStoreName=DiagcMgrNtcMap  InitialValue=[0 0 0 0 0 0 0 0 0 0 0 0 0 0 0 0 0 0 0 0 0 0 0 0 0 0 0 0 0 0 0 0 0 0 0 0 0 0 0 0 0 0 0 0 0 0 0 0 0 0 0 0 0 0 0 0 0 0 0 0 0 0 0 0 0 0 0 0 0 0 0 0 0 0 0 0 0 0 0 0 0 0 0 0 0 0 0 0 0 0 0 0 0 0 0 0 0 0 0 0 0 0 0 0 0 0 0 0 0 0 0 0 0 0 0 0 0 0 0 0 0 0 0 0 0 0 0 0 0 0 0 0 0 0 0 0 0 0 0 0 0 0 0 0 0 0 0 0 0 0 0 0 0 0 0 0 0 0 0 0 0 0 0 0 0 0 0 0 0 0 0 0 0 0 0 0 0 0 0 0 0 0 0 0 0 0 0 0 0 0 0 0 0 0 0 0 0 0 0 0 0 0 0 0 0 0 0 0 0 0 0 0 0 0 0 0 0 0 0 0 0 0 0 0 0 0 0 0 0 0 0 0 0 0 0 0 0 0 0 0 0 0 0 0 0 0 0 0 0 0 0 0 0 0 0 0 0 0 0 0 0 0 0 0 0 0 0 0 0 0 0 0 0 0 0 0 0 0 0 0 0 0 0 0 0 0 0 0 0 0 0 0 0 0 0 0 0 0 0 0 0 0 0 0 0 0 0 0 0 0 0 0 0 0 0 0 0 0 0 0 0 0 0 0 0 0 0 0 0 0 0 0 0 0 0 0 0 0 0 0 0 0 0 0 0 0 0 0 0 0 0 0 0 0 0 0 0 0 0 0 0 0 0 0 0 0 0 0 0 0 0 0 0 0 0 0 0 0 0 0 0 0 0 0 0 0 0 0 0 0 0 0 0 0 0 0 0 0 0 0 0 0 0 0 0 0 0 0 0 0 0 0 0 0 0 0 0 0 0 0 0 0 0 0 0 0 0 0 0 0 0 0 0 0 0 0 0 0 0 0 0 0 0 0 0 0 0 0 0 0 0 0 0 0 0 0 0 0 0 0 0 0 0 0 0 0 0 0 0 0 0 0 0 0 0 0 0 0 0 0 0 0 0 0 0 0 0 0 0 0 0 0 0 0 0 0 0 0 0 0 0 0 0 0 0 0 0 0 0 0 0 0]  OutDataTypeStr=Bus: NtcMapRec2
      settings: AttributesFormatString=%<Description>
  "GetNtcActvCore " : Subsystem  RequirementInfo={} %GIDa_04448c3d_38d3_46e4_b172_adc3c24b63ba
      settings: AttributesFormatString=%<Description>
  "GetNtcQlfrStsCore " : Subsystem  RequirementInfo={} %GIDa_01811d8f_602c_4edc_a6c9_bf2cc3d3a807
  GetNtcStsCore : Subsystem  RequirementInfo={} %GIDa_71884bca_182b_4f84_8287_d1491f58d6bb
  NvM Set Ram Block Status Block Changed : DataStoreMemory  DataStoreName=NvMSRBS_BlockChanged  OutDataTypeStr=uint8
  NvM: Diagnostic Manager Power Down Fault Array : DataStoreMemory  RequirementInfo="{'linktype_rmi_doors' '0000c474 (/ESG Group/FDD Module Requirements/EA4 Specific/ES101A_DiagcMgr)' '#ES101A_213' 'true' 'REQ:  ES101A_213' '' } %GIDa_715eabb4_bc85_46f0_b853_2ddaaa9c03a0"  DataStoreName=DiagcMgrNtcFltAry  InitialValue=[0 0 0 0 0 0 0 0 0 0 0 0 0 0 0 0 0 0 0 0]  OutDataTypeStr=Bus: NtcFltInfoRec1  Dimensions=20  StateMustResolveToSignalObject=on
  NvM: Snapshot Data Array : DataStoreMemory  RequirementInfo="{'linktype_rmi_doors' '0000c474 (/ESG Group/FDD Module Requirements/EA4 Specific/ES101A_DiagcMgr)' '#ES101A_326' 'true' 'REQ:  ES101A_326' '' } %GIDa_607aeee7_d0c7_4a84_a8c5_94c2db8a3562"  DataStoreName=SnpshtDataAry  InitialValue=[0 0 0 0 0 0 0 0 0 0 0 0 0 0 0 0 0 0 0 0]  OutDataTypeStr=Bus: SnpshtDataRec1  Dimensions=20  StateMustResolveToSignalObject=on
  PIM: Clear Diagnsotics Flag : DataStoreMemory  DataStoreName=ClrDiagcFlg  OutDataTypeStr=uint8  StateMustResolveToSignalObject=on
  PIM: DTC Enable Status : DataStoreMemory  DataStoreName=DtcEnaSts  OutDataTypeStr=uint16  StateMustResolveToSignalObject=on
  PIM: DTC Index Previous Status : DataStoreMemory  DataStoreName=DtcIdxPrevSts  InitialValue=[0 0 0 0 0 0 0 0 0 0 0 0 0 0 0 0 0 0 0 0 0 0 0 0 0 0 0 0 0 0 0 0 0 0 0 0 0 0 0 0 0 0 0 0 0 0 0 0 0 0 0 0 0 0 0 0 0 0 0 0 0 0 0 0 0 0 0 0 0 0 0 0 0 0 0 0 0 0 0 0 0 0 0 0 0 0 0 0 0 0 0 0 0 0 0 0 0 0 0 0 0 0 0 0 0 0 0 0 0 0 0 0 0 0 0 0 0 0 0 0 0 0 0 0 0 0 0 0 0 0 0 0 0 0 0 0 0 0 0 0 0 0 0 0 0 0 0 0 0 0 0 0 0 0 0 0 0 0 0 0 0 0 0 0 0 0 0 0 0 0 0 0 0 0 0 0 0 0 0 0 0 0 0 0 0 0 0 0 0 0 0 0 0 0 0 0 0 0 0 0 0 0 0 0 0 0 0 0 0 0 0 0 0 0 0 0 0 0 0 0 0 0 0 0 0 0 0 0 0 0 0 0 0 0 0 0 0 0 0 0 0 0 0 0 0 0 0 0 0 0 0 0 0 0 0 0]  OutDataTypeStr=uint8  StateMustResolveToSignalObject=on
  PIM: Previous Clear DTC Flag : DataStoreMemory  DataStoreName=PrevClrDtcFlg  OutDataTypeStr=uint8  StateMustResolveToSignalObject=on
  ProxySetNtcData : Constant  Value=ProxySetNtcData
  ReadNtcFltAry : Subsystem  RequirementInfo="{'linktype_rmi_doors' '0000c474 (/ESG Group/FDD Module Requirements/EA4 Specific/ES101A_DiagcMgr)' '#ES101A_248' 'true' 'REQ:  ES101A_248' '' ; 'linktype_rmi_doors' '0000c474 (/ESG Group/FDD Module Requirements/EA4 Specific/ES101A_DiagcMgr)' '#ES101A_249' 'true' 'REQ:  ES101A_249' '' ; 'linktype_rmi_doors' '0000c474 (/ESG Group/FDD Module Requirements/EA4 Specific/ES101A_DiagcMgr)' '#ES101A_217' 'true' 'REQ:  ES101A_217' '' ; 'linktype_rmi_doors' '0000c474 (/ESG Group/FDD Module Requirements/EA4 Specific/ES101A_DiagcMgr)' '#ES101A_211' 'true' 'REQ:  ES101A_211' '' } %GIDa_5bfe570e_f6ed_4b10_a6e9_18fee0ad166c"
  ReadNtcInfoAndDebCntr : Subsystem  RequirementInfo="{'linktype_rmi_doors' '0000c474 (/ESG Group/FDD Module Requirements/EA4 Specific/ES101A_DiagcMgr)' '#ES101A_343' 'true' 'REQ:  ES101A_343' '' } %GIDa_724a722c_beca_4e37_86ed_9254eb616607"
  ReadSnpshtData : Subsystem  RequirementInfo="{'linktype_rmi_doors' '0000c474 (/ESG Group/FDD Module Requirements/EA4 Specific/ES101A_DiagcMgr)' '#ES101A_333' 'true' 'REQ:  ES101A_333' '' } %GIDa_b2bebb6f_a79b_43d4_9b5f_3c33a2736d32"
  RestoreNtcFltAryDft : Subsystem  Description=Non RTE Server Runnable  RequirementInfo="{'linktype_rmi_doors' '0000c474 (/ESG Group/FDD Module Requirements/EA4 Specific/ES101A_DiagcMgr)' '#ES101A_246' 'true' 'REQ:  ES101A_246' '' } %GIDa_03e13866_7d05_49c0_85fb_045f5a6b8ea2"
      settings: AttributesFormatString=%<Description>
  RestoreSnpshtAryDft : Subsystem  Description=Non RTE Server Runnable  RequirementInfo="{'linktype_rmi_doors' '0000c474 (/ESG Group/FDD Module Requirements/EA4 Specific/ES101A_DiagcMgr)' '#ES101A_332' 'true' 'REQ:  ES101A_332' '' } %GIDa_42553798_7ae5_4c83_a272_46d073e974ec"
      settings: AttributesFormatString=%<Description>
  SetNtcStsCore : Subsystem  RequirementInfo="{'linktype_rmi_doors' '0000c474 (/ESG Group/FDD Module Requirements/EA4 Specific/ES101A_DiagcMgr)' '#ES101A_167' 'true' 'REQ:  ES101A_167' '' ; 'linktype_rmi_doors' '0000c474 (/ESG Group/FDD Module Requirements/EA4 Specific/ES101A_DiagcMgr)' '#ES101A_67' 'true' 'REQ:  ES101A_67' '' ; 'linktype_rmi_doors' '0000c474 (/ESG Group/FDD Module Requirements/EA4 Specific/ES101A_DiagcMgr)' '#ES101A_91' 'true' 'REQ:  ES101A_91' '' } %GIDa_0a973d9a_1491_4fd9_85bd_a83db0e93c58"
  UpdDtcEnaCdn : Subsystem  Description=|  RequirementInfo={} %GIDa_31cda807_ea73_4f05_ad8d_6edfca28fdc0
      | The design assumes that this server function will not re-entrant.
      | It is assumed that only the BSWM will call this function.
      | This is the reason why we don't have this function as an "exclusive area".
      settings: AttributesFormatString=%<Description>
  "NtcInfo_ArgOut " : Outport
  NtcQlfr_ArgOut : Outport  Port=2
  NtcActv_ArgOut : Outport  Port=3
  NtcInfoSts_ArgOut : Outport  Port=4
  "DiagcData_ArgOut " : Outport  Port=5
  "ProxySetNtcData_ArgOut " : Outport  Port=6
  "NtcInfoDebCntr_ArgOut " : Outport  Port=7
  ProxySetNtcData_ArgOut : Outport  Port=8
  DiagcData_ArgOut : Outport  Port=9
  SetNtcStsCore_StdRtn : Outport  Port=10
  DiagcMgrReadFltInfo_ArgOut : Outport  Port=11
  SysDiRampRate : Outport  RequirementInfo={} %GIDa_c741bd04_a277_4637_b269_8ad7c88aafb3  Port=12
  SysDiMotTqCmdSca : Outport  RequirementInfo={} %GIDa_4dfe7251_b00a_4f03_9c43_b194a34236fb  Port=13
  SysStFltOutpReqDi : Outport  RequirementInfo={} %GIDa_ab910246_4f00_4eec_b765_0ada87af3f7b  Port=14
  DiagcStsLimdTPrfmnc : Outport  RequirementInfo={} %GIDa_8dd0be71_117e_49ff_9403_16ceb7bdcd0f  Port=15
  DiagcStsIvtr1Inactv : Outport  RequirementInfo={} %GIDa_84e2b0e7_a62f_4137_ac4a_536040590d20  Port=16
  DiagcStsIvtr2Inactv : Outport  RequirementInfo={} %GIDa_9a3644ce_0917_46d4_99f2_f91c8dc1c034  Port=17
  DiagcStsDftHwAg : Outport  RequirementInfo={} %GIDa_236e619f_ef63_41c2_946d_b85ab965e504  Port=18
  DiagcStsDftVehSpd : Outport  RequirementInfo={} %GIDa_4abfde6b_766b_4ce0_bb85_4f0699e22aec  Port=19
  DiagcStsDftHwAgSerlComExprtVal : Outport  RequirementInfo={} %GIDa_8ae6f221_8731_49da_a722_aa274fb021b6  Port=20
  DiagcStsWhlImbRejctnDi : Outport  RequirementInfo={} %GIDa_28fb3d72_5c82_4b15_b3a1_adacc1fecf42  Port=21
  DiagcStsCtrldShtDwnFltPrsnt : Outport  RequirementInfo={} %GIDa_06bebeed_8d2e_4596_be4d_9fb42201984c  Port=22
  ClrDiagcFlgProxy : Outport  Port=23
  NtcInfoAry_ArgOut : Outport  Port=24
  ReadSnpshtAry_ArgOut : Outport  Port=25
  NtcInfo_ArgOut : Outport  Port=26
  DebCntr_ArgOut : Outport  Port=27
  wires:
  SetNtcStsCore/2(SetNtcStsCore_StdRtn) -> SetNtcStsCore_StdRtn/1
  call_SetNtcStsCore/1 -> SetNtcStsCore/Trigger
  DebStep_ArgIn/1 -> SetNtcStsCore/4(DebStep_ArgIn)
  NtcStInfo_ArgIn/1 -> SetNtcStsCore/2(NtcStInfo_ArgIn)
  NtcSts_ArgIn/1 -> SetNtcStsCore/3(NtcSts_ArgIn)
  call_DiagcMgrIninCore/1 -> DiagcMgrIninCore/Trigger
  call_GetNtcQlfrStsCore/1 -> "GetNtcQlfrStsCore "/Trigger
  call_GetNtcActvCore/1 -> "GetNtcActvCore "/Trigger
  call_GetNtcStsCore/1 -> GetNtcStsCore/Trigger
  GetNtcStsCore/1(NtcInfoSts_ArgOut) -> NtcInfoSts_ArgOut/1
  call_ClrAllDiagc/1 -> ClrAllDiagc/Trigger
  SysSt/1 -> SetNtcStsCore/5(SysSt)
  MfgEnaSt/1 -> SetNtcStsCore/6(MfgEnaSt)
  MfgDiagcInhb/1 -> SetNtcStsCore/7(MfgDiagcInhb)
  call_DiagcMgrPwrDwn/1 -> DiagcMgrPwrDwn/Trigger
  "GetNtcActvCore "/1(NtcActv_ArgOut) -> NtcActv_ArgOut/1
  "GetNtcQlfrStsCore "/1(NtcQlfr_ArgOut) -> NtcQlfr_ArgOut/1
  call_ReadNtcFltAry/1 -> ReadNtcFltAry/Trigger
  ReadNtcFltAry/1(DiagcMgrReadFltInfo_ArgOut) -> DiagcMgrReadFltInfo_ArgOut/1
  call_DiagcMgrPer1/1 -> DiagcMgrPer1/Trigger
  DiagcMgrPer1/6(DiagcStsIvtr2Inactv) -> DiagcStsIvtr2Inactv/1
  DiagcMgrPer1/4(DiagcStsLimdTPrfmnc) -> DiagcStsLimdTPrfmnc/1
  DiagcMgrPer1/3(SysStFltOutpReqDi) -> SysStFltOutpReqDi/1
  DiagcMgrPer1/1(SysDiRampRate) -> SysDiRampRate/1
  DiagcMgrPer1/5(DiagcStsIvtr1Inactv) -> DiagcStsIvtr1Inactv/1
  DiagcMgrPer1/2(SysDiMotTqCmdSca) -> SysDiMotTqCmdSca/1
  DiagcMgrPer1/7(DiagcStsDftHwAg) -> DiagcStsDftHwAg/1
  DiagcMgrPer1/8(DiagcStsDftVehSpd) -> DiagcStsDftVehSpd/1
  DiagcMgrPer1/9(DiagcStsDftHwAgSerlComExprtVal) -> DiagcStsDftHwAgSerlComExprtVal/1
  DiagcMgrPer1/10(DiagcStsWhlImbRejctnDi) -> DiagcStsWhlImbRejctnDi/1
  DiagcMgrPer1/11(DiagcStsCtrldShtDwnFltPrsnt) -> DiagcStsCtrldShtDwnFltPrsnt/1
  NtcInfo_ArgIn/1 -> SetNtcStsCore/10(NtcInfo_ArgIn)
  DiagcData_ArgIn/1 -> SetNtcStsCore/8(DiagcData_ArgIn)
  ProxySetNtcData_ArgIn/1 -> SetNtcStsCore/9(ProxySetNtcData_ArgIn)
  SetNtcStsCore/1("NtcInfo_ArgOut ") -> "NtcInfo_ArgOut "/1
  call_RestoreNtcFltAryDft/1 -> RestoreNtcFltAryDft/Trigger
  SetNtcStsCore/3("DiagcData_ArgOut ") -> "DiagcData_ArgOut "/1
  SetNtcStsCore/4("ProxySetNtcData_ArgOut ") -> "ProxySetNtcData_ArgOut "/1
  ApplIdx_ArgIn/1 -> DiagcMgrIninCore/1(AppIdx_ArgIn)
  DiagcMgrIninCore/1(ProxySetNtcData_ArgOut) -> ProxySetNtcData_ArgOut/1
  DiagcMgrIninCore/2(DiagcData_ArgOut) -> DiagcData_ArgOut/1
  DiagcMgrIninCore/3(NtcInfoAry_ArgOut) -> NtcInfoAry_ArgOut/1
  NtcInfoArySize_ArgIn/1 -> DiagcMgrIninCore/2(NtcInfoArySize)
  NtcInfoDebCntr_ArgIn/1 -> SetNtcStsCore/11(NtcInfoDebCntr_ArgIn)
  SetNtcStsCore/5("NtcInfoDebCntr_ArgOut ") -> "NtcInfoDebCntr_ArgOut "/1
  NtcInfoAry_ArgIn/1 -> DiagcMgrIninCore/3(NtcInfoAry_ArgIn)
  ProxySetNtcData/1 -> DiagcMgrIninCore/5(ProxySetNtcData)
  DiagcData/1 -> DiagcMgrIninCore/4(DiagcData)
  call_DiagcMgrPer2/1 -> DiagcMgrPer2/Trigger
  call_UpdDtcEnaCdn/1 -> UpdDtcEnaCdn/Trigger
  DtcEnaCdnSts_ArgIn/1 -> UpdDtcEnaCdn/1(DtcEnaCdnSts_ArgIn)
  DtcEnaCdnId_ArgIn/1 -> UpdDtcEnaCdn/2(DtcEnaCdnId_ArgIn)
  ClrAllDiagc/1(ClrDiagcFlgProxy) -> ClrDiagcFlgProxy/1
  call_ClrSnpshtData/1 -> ClrSnpshtData/Trigger
  call_ReadSnpshtData/1 -> ReadSnpshtData/Trigger
  ReadSnpshtData/1(ReadSnpshtAry_ArgOut) -> ReadSnpshtAry_ArgOut/1
  IgnCntr/1 -> SetNtcStsCore/12(IgnCntr)
  RegInBRAMDAT1/1 -> SetNtcStsCore/13(RegInBRAMDAT1)
  HwTq/1 -> SetNtcStsCore/14(HwTq)
  MotTqCmdMrfScad/1 -> SetNtcStsCore/15(MotTqCmdMrfScad)
  BrdgVltg/1 -> SetNtcStsCore/16(BrdgVltg)
  EcuTFild/1 -> SetNtcStsCore/17(EcuTFild)
  VehSpd/1 -> SetNtcStsCore/18(VehSpd)
  NtcNr_ArgIn/1 -> GetNtcStsCore/1(NtcNr_ArgIn), "GetNtcActvCore "/1(NtcNr_ArgIn), "GetNtcQlfrStsCore "/1(NtcNr_ArgIn), ReadNtcInfoAndDebCntr/1(NtcNr_ArgIn), SetNtcStsCore/1(NtcNr_ArgIn)
  call_GetNtcInfoCore/1 -> ReadNtcInfoAndDebCntr/Trigger
  ReadNtcInfoAndDebCntr/1(NtcInfo_ArgOut) -> NtcInfo_ArgOut/1
  ReadNtcInfoAndDebCntr/2(DebCntr_ArgOut) -> DebCntr_ArgOut/1
  call_RestoreSnpShtAryDft/1 -> RestoreSnpshtAryDft/Trigger

== system ES101A_DiagcMgr/DiagcMgr/ClrAllDiagc ==
  Function : TriggerPort  TriggerType=function-call
  CopyRight2 : Subsystem  Description=|  mask(Copyright Information){none=on}
      | Copyright info block.                                               
      |                                                                     
      | Place copyright information at the top of every subsystem in design.
      mask prompts: none "No parameters"
      mask help: Place copyright information at the top of every subsystem in design.
      mask Display:
      | NxtrConf = 'Nexteer Confidential';
      | 
      | sys = bdroot; %handle for the current model ("system")
      | first = get_param(sys,'Created');
      | first = first(end-3:end);  %year is last four digits
      | 
      | last = get_param(sys,'LastModifiedDate');
      | if isempty(last)
      |     last = datestr(now,'yyyy');
      | else
      |     last = last(end-3:end);
      | end
      | 
      | if strcmp(first,last)
      |     fprintf('%s -- Copyright %s Nexteer',NxtrConf,first)
      | else
      |     fprintf('%s -- %s%s- %s Nexteer',NxtrConf,char(169),first,last)
      | end
  Data Store Read : DataStoreRead  DataStoreName=ClrDiagcFlg
  Data Store Write : DataStoreWrite  DataStoreName=ClrDiagcFlg
  If : If  IfExpression=u1 == 1
  If Action Subsystem : Subsystem  TreatAsAtomicUnit=on
  If Action Subsystem1 : Subsystem  TreatAsAtomicUnit=on
  Merge : Merge
  ClrDiagcFlgProxy : Outport  InitialOutput=1
  wires:
  Data Store Read/1 -> If/1
  If/1 -> If Action Subsystem/Action
  If/2 -> If Action Subsystem1/Action
  Merge/1 -> ClrDiagcFlgProxy/1, Data Store Write/1
  If Action Subsystem/1(ClrDiagcFlg) -> Merge/1
  If Action Subsystem1/1(ClrDiagcFlg) -> Merge/2
